simulink model "dc_motor_models"  (R2017b)
settings: Solver=FixedStepAuto  StartTime=0.0  StopTime=20  FixedStep=0.001  RelTol=1e-3
values from neighbouring files (symbols this model uses):
  Aa = [0 1 0; 0 0 1; 0 -(R*k_f+k_m*k_e)/(L*J) -(L*k_f+R*J)/(L*J)]    [dc_motor_parameters.m]
  Av = [0 1; -(R*k_f+k_m*k_e)/(L*J) -(L*k_f+R*J)/(L*J)]    [dc_motor_parameters.m]
  Ba = [0; 0; k_m/(L*J)]    [dc_motor_parameters.m]
  Bv = [0; k_m/(L*J)]    [dc_motor_parameters.m]
  Ca = [1 0 0]    [dc_motor_parameters.m]
  Cv = [1 0]    [dc_motor_parameters.m]
  J = J_d+J_m    (= 0.1)    [dc_motor_parameters.m]
  K_D = 1/R    (= 1)    [dc_motor_parameters.m]
  k_e = 0.1    [dc_motor_parameters.m]
  k_f = 0.2    [dc_motor_parameters.m]
  k_m = 0.5    [dc_motor_parameters.m]
  L = 1    [dc_motor_parameters.m]
  M_d = 0    [dc_motor_parameters.m]
  R = 1    [dc_motor_parameters.m]
  T = L/R    (= 1)    [dc_motor_parameters.m]
settings Model: Creator=Алексей  LastModifiedBy=alexe
settings CodeAppCC: StateflowObjectComments=on

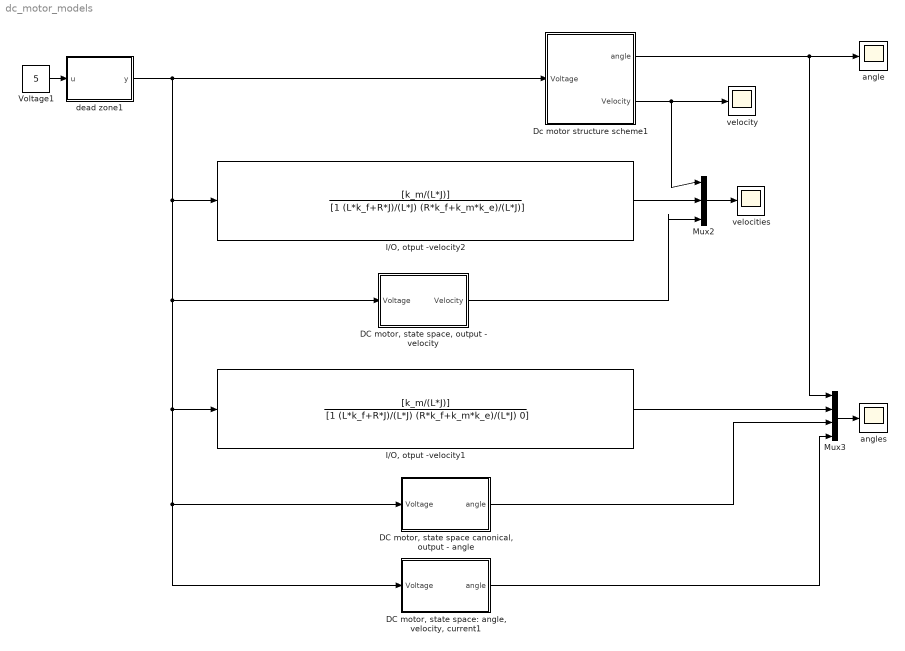
== system dc_motor_models ==
  "DC motor, state space canonical, output - angle" : Subsystem
  "DC motor, state space, output - velocity" : Subsystem
  "DC motor, state space: angle, velocity, current1" : Subsystem
  Dc motor structure scheme1 : Subsystem
  "I/O, otput -velocity1" : TransferFcn  Numerator=[k_m/(L*J)]  Denominator=[1 (L*k_f+R*J)/(L*J) (R*k_f+k_m*k_e)/(L*J) 0]
  "I/O, otput -velocity2" : TransferFcn  Numerator=[k_m/(L*J)]  Denominator=[1 (L*k_f+R*J)/(L*J) (R*k_f+k_m*k_e)/(L*J)]
  Mux2 : Mux  Inputs=3
  Mux3 : Mux
  Voltage1 : Constant  Value=5
  angle : Scope
  angles : Scope
  dead zone1 : MATLAB Function  TreatAsAtomicUnit=on
  velocities : Scope
  velocity : Scope
  wires:
  Voltage1/1 -> dead zone1/1(u)
  Dc motor structure scheme1/1(angle) -> Mux3/1, angle/1
  Dc motor structure scheme1/2(Velocity) -> Mux2/1, velocity/1
  Mux2/1 -> velocities/1
  "I/O, otput -velocity2"/1 -> Mux2/2
  "DC motor, state space, output - velocity"/1(Velocity) -> Mux2/3
  "I/O, otput -velocity1"/1 -> Mux3/2
  Mux3/1 -> angles/1
  "DC motor, state space canonical, output - angle"/1(angle) -> Mux3/3
  "DC motor, state space: angle, velocity, current1"/1(angle) -> Mux3/4
  dead zone1/1(y) -> Dc motor structure scheme1/1(Voltage), "DC motor, state space canonical, output - angle"/1(Voltage), "DC motor, state space: angle, velocity, current1"/1(Voltage), "I/O, otput -velocity1"/1, "DC motor, state space, output - velocity"/1(Voltage), "I/O, otput -velocity2"/1

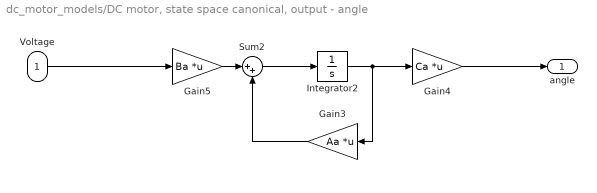
== system dc_motor_models/DC motor, state space canonical, output - angle ==
  Voltage : Inport
  Gain3 : Gain  Gain=Aa  Multiplication=Matrix(K*u) (u vector)
  Gain4 : Gain  Gain=Ca  Multiplication=Matrix(K*u) (u vector)
  Gain5 : Gain  Gain=Ba  Multiplication=Matrix(K*u) (u vector)
  Integrator2 : Integrator
  Sum2 : Sum  Inputs=|++
  angle : Outport
  wires:
  Voltage/1 -> Gain5/1
  Gain5/1 -> Sum2/1
  Gain3/1 -> Sum2/2
  Gain4/1 -> angle/1
  Integrator2/1 -> Gain3/1, Gain4/1
  Sum2/1 -> Integrator2/1

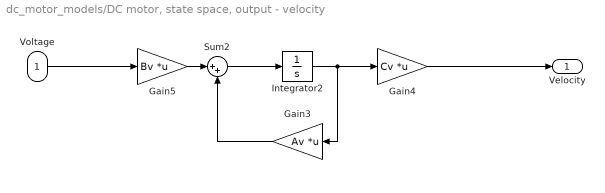
== system dc_motor_models/DC motor, state space, output - velocity ==
  Voltage : Inport
  Gain3 : Gain  Gain=Av  Multiplication=Matrix(K*u) (u vector)
  Gain4 : Gain  Gain=Cv  Multiplication=Matrix(K*u) (u vector)
  Gain5 : Gain  Gain=Bv  Multiplication=Matrix(K*u) (u vector)
  Integrator2 : Integrator
  Sum2 : Sum  Inputs=|++
  Velocity : Outport
  wires:
  Sum2/1 -> Integrator2/1
  Integrator2/1 -> Gain4/1, Gain3/1
  Gain4/1 -> Velocity/1
  Gain3/1 -> Sum2/2
  Gain5/1 -> Sum2/1
  Voltage/1 -> Gain5/1

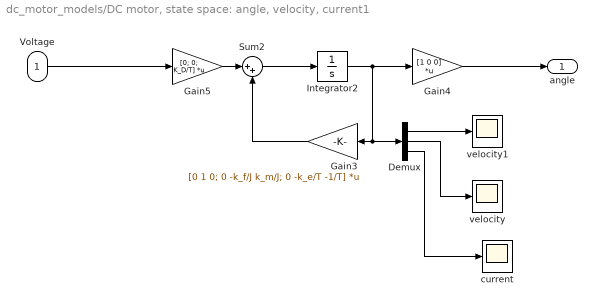
== system dc_motor_models/DC motor, state space: angle, velocity, current1 ==
  Voltage : Inport
  Demux : Demux  Outputs=3
  Gain3 : Gain  Gain=[0 1 0; 0 -k_f/J k_m/J; 0 -k_e/T -1/T]  Multiplication=Matrix(K*u) (u vector)
  Gain4 : Gain  Gain=[1 0 0]  Multiplication=Matrix(K*u) (u vector)
  Gain5 : Gain  Gain=[0; 0; K_D/T]  Multiplication=Matrix(K*u) (u vector)
  Integrator2 : Integrator
  Sum2 : Sum  Inputs=|++
  current : Scope
  velocity : Scope
  velocity1 : Scope
  angle : Outport
  wires:
  Demux/3 -> current/1
  Demux/1 -> velocity1/1
  Demux/2 -> velocity/1
  Sum2/1 -> Integrator2/1
  Integrator2/1 -> Gain4/1, Gain3/1, Demux/1
  Gain4/1 -> angle/1
  Gain3/1 -> Sum2/2
  Gain5/1 -> Sum2/1
  Voltage/1 -> Gain5/1

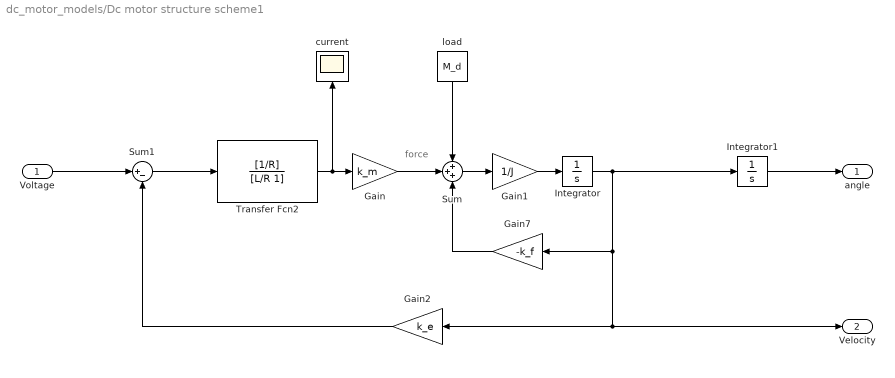
== system dc_motor_models/Dc motor structure scheme1 ==
  note: force
  Voltage : Inport
  Gain : Gain  Gain=k_m
  Gain1 : Gain  Gain=1/J
  Gain2 : Gain  Gain=k_e
  Gain7 : Gain  Gain=-k_f
  Integrator : Integrator
  Integrator1 : Integrator
  Sum : Sum  Inputs=+++
  Sum1 : Sum  Inputs=|+-
  Transfer Fcn2 : TransferFcn  Numerator=[1/R]  Denominator=[L/R 1]
  current : Scope
  load : Constant  Value=M_d
  angle : Outport
  Velocity : Outport  Port=2
  wires:
  load/1 -> Sum/1
  Integrator/1 -> Integrator1/1, Gain2/1, Velocity/1, Gain7/1
  Sum/1 -> Gain1/1
  Voltage/1 -> Sum1/1
  Sum1/1 -> Transfer Fcn2/1
  Integrator1/1 -> angle/1
  Gain1/1 -> Integrator/1
  Gain2/1 -> Sum1/2
  Gain/1 -> Sum/2
  Transfer Fcn2/1 -> Gain/1, current/1
  Gain7/1 -> Sum/3

== matlab function dc_motor_models/dead zone1 ==
  data: u input; y output
function y = fcn(u)
if abs(u)<3
    y=0;
else
    if abs(u)>5
        y=sign(u)*5;
    else
        y=u;
    end
end
